simulink model "dyskretny_nieliniowy_model_dynamiczny"  (R2022b)
settings: Solver=VariableStepAuto  StartTime=0.0  StopTime=100  RelTol=1e-3
values from neighbouring files (symbols this model uses):
  a0 = 0.00185185    [Projekt1.m]    (also in transmitancja_dyskretna.m = data.a0; wykresy_char_stat_nlin.m = data.a0; wykresy_char_stat_zlin.m = data.a0)
  a1 = 0.0462963    [Projekt1.m]    (also in transmitancja_dyskretna.m = data.a1; wykresy_char_stat_nlin.m = data.a1; wykresy_char_stat_zlin.m = data.a1)
  a2 = 0.377778    [Projekt1.m]    (also in transmitancja_dyskretna.m = data.a2; wykresy_char_stat_nlin.m = data.a2; wykresy_char_stat_zlin.m = data.a2)
  alpha1 = 0.4    [Projekt1.m]    (also in transmitancja_dyskretna.m = data.alpha1; wykresy_char_stat_nlin.m = data.alpha1; wykresy_char_stat_zlin.m = data.alpha1)
  alpha2 = 0.55    [Projekt1.m]    (also in transmitancja_dyskretna.m = data.alpha2; wykresy_char_stat_nlin.m = data.alpha2; wykresy_char_stat_zlin.m = data.alpha2)
  alpha3 = -0.92    [Projekt1.m]    (also in transmitancja_dyskretna.m = data.alpha3; wykresy_char_stat_nlin.m = data.alpha3; wykresy_char_stat_zlin.m = data.alpha3)
  alpha4 = 0.53    [Projekt1.m]    (also in transmitancja_dyskretna.m = data.alpha4; wykresy_char_stat_nlin.m = data.alpha4; wykresy_char_stat_zlin.m = data.alpha4)
  b0 = 0.00333333    [Projekt1.m]    (also in transmitancja_dyskretna.m = data.b0; wykresy_char_stat_nlin.m = data.b0; wykresy_char_stat_zlin.m = data.b0)
  T = T_sim(i)    [Projekt1.m]    (also in wykresy_char_dyn_dys.m)
  t_u_step_sim = 1    [Projekt1.m]    (also in wykresy_char_dyn_dys.m)
  u_step_sim = 1    [Projekt1.m]    (also in wykresy_char_dyn_dys.m)
settings Model: Creator=pioro  LastModifiedBy=pioro

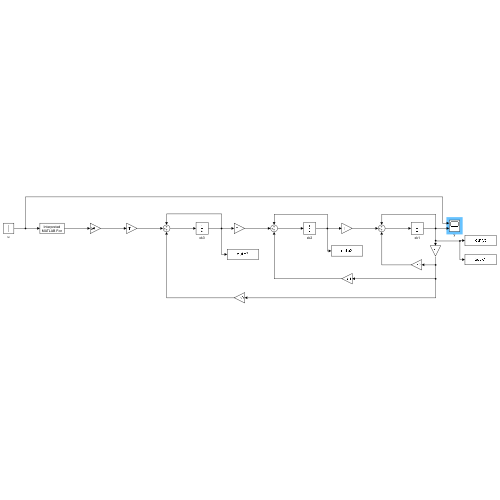
[thumbnail: Simulink's stored preview of the top-level diagram]
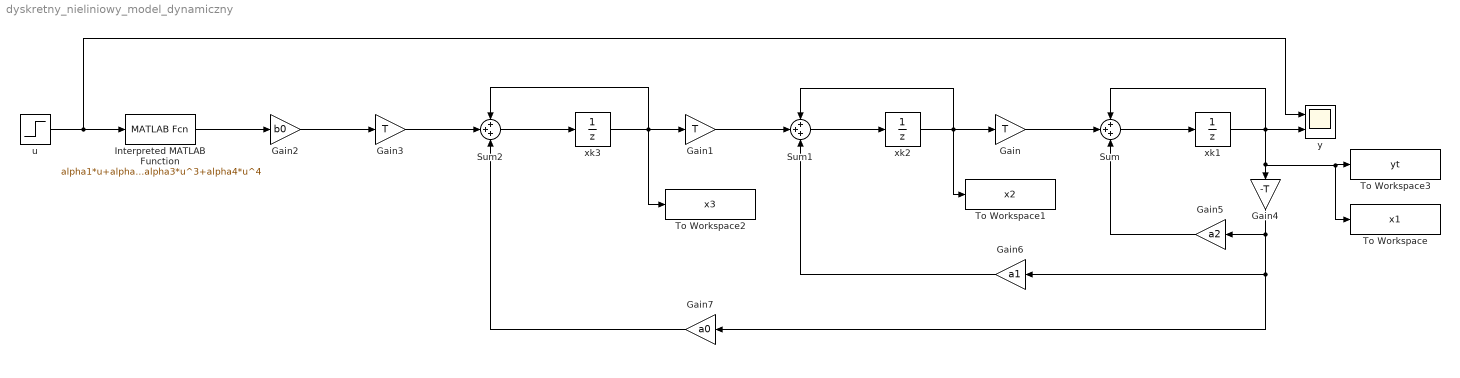
== system dyskretny_nieliniowy_model_dynamiczny ==
  Gain : Gain  Gain=T
  Gain1 : Gain  Gain=T
  Gain2 : Gain  Gain=b0
  Gain3 : Gain  Gain=T
  Gain4 : Gain  Gain=-T
  Gain5 : Gain  Gain=a2
  Gain6 : Gain  Gain=a1
  Gain7 : Gain  Gain=a0
  Interpreted MATLAB Function : MATLABFcn  MATLABFcn=alpha1*u+alpha2*u^2+alpha3*u^3+alpha4*u^4
  Sum : Sum  Inputs=+++
  Sum1 : Sum  Inputs=+++
  Sum2 : Sum  Inputs=+++
  To Workspace : ToWorkspace  VariableName=x1  SaveFormat=Timeseries  SampleTime=-1
  To Workspace1 : ToWorkspace  VariableName=x2  SaveFormat=Timeseries  SampleTime=-1
  To Workspace2 : ToWorkspace  VariableName=x3  SaveFormat=Timeseries  SampleTime=-1
  To Workspace3 : ToWorkspace  VariableName=yt  SaveFormat=Timeseries  SampleTime=-1
  u : Step  Time=t_u_step_sim  After=u_step_sim  SampleTime=0
  xk1 : UnitDelay  SampleTime=T  HasFrameUpgradeWarning=on
  xk2 : UnitDelay  SampleTime=T  HasFrameUpgradeWarning=on
  xk3 : UnitDelay  SampleTime=T  HasFrameUpgradeWarning=on
  y : Scope  NumInputPorts=2
  wires:
  Sum/1 -> xk1/1
  Gain/1 -> Sum/2
  Gain5/1 -> Sum/3
  Gain1/1 -> Sum1/2
  xk3/1 -> To Workspace2/1, Gain1/1, Sum2/1
  Sum1/1 -> xk2/1
  Gain6/1 -> Sum1/3
  Gain7/1 -> Sum2/3
  Sum2/1 -> xk3/1
  Gain2/1 -> Gain3/1
  Interpreted MATLAB Function/1 -> Gain2/1
  Gain3/1 -> Sum2/2
  xk1/1 -> Sum/1, To Workspace3/1, To Workspace/1, Gain4/1, y/2
  u/1 -> Interpreted MATLAB Function/1, y/1
  Gain4/1 -> Gain5/1, Gain7/1, Gain6/1
  xk2/1 -> Sum1/1, To Workspace1/1, Gain/1
